simulink model "Schimmel_Evan_lab_4_model_single"  (R2020b)
settings: Solver=VariableStepAuto  StartTime=0.0  StopTime=tf  MaxStep=maxstep  RelTol=tol  AbsTol=tol
values from neighbouring files (symbols this model uses):
  C = mp*lpcg+mw*lwcg    (= 0.01745975)    [Schimmel_Evan_lab_4_script_double.m]    (also in Schimmel_Evan_lab_4_script_single.m)
  J = ((mp*lp^2)/12)+mp*(lpcg^2)+(1/2)*mw*((dw/2)^2)+mw*(lwcg^2)    (= 0.004070351125)    [Schimmel_Evan_lab_4_script_double.m]    (also in Schimmel_Evan_lab_4_script_single.m)
  k = g*(mp*lpcg+mw*lwcg)    (= 0.1712801475)    [Schimmel_Evan_lab_4_script_double.m]    (also in Schimmel_Evan_lab_4_script_single.m)
  omega0 = 0    [Schimmel_Evan_lab_4_script_double.m]    (also in Schimmel_Evan_lab_4_script_single.m)
  theta0 = 0    [Schimmel_Evan_lab_4_script_double.m]    (also in Schimmel_Evan_lab_4_script_single.m)
settings Model: Creator=schimmer  LastModifiedBy=schimmer
settings DataIOCC: SaveOutput=off  SignalLogging=off  DSMLogging=off  SaveTime=off  ReturnWorkspaceOutputs=off

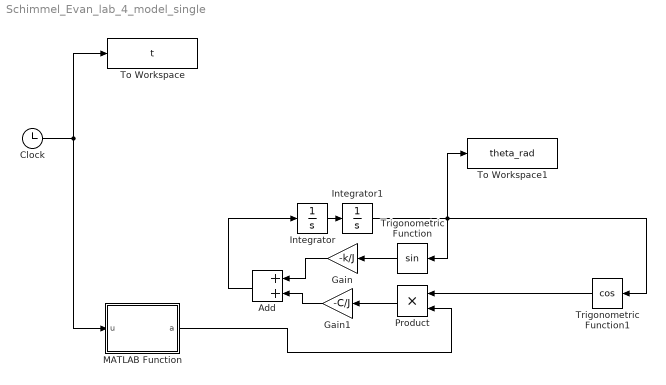
== system Schimmel_Evan_lab_4_model_single ==
  Add : Sum
  Clock : Clock
  Gain : Gain  Gain=-k/J
  Gain1 : Gain  Gain=-C/J
  Integrator : Integrator  InitialCondition=omega0
  Integrator1 : Integrator  InitialCondition=theta0
  MATLAB Function : MATLAB Function  TreatAsAtomicUnit=on
  Product : Product
  To Workspace : ToWorkspace  VariableName=t  SampleTime=-1
  To Workspace1 : ToWorkspace  VariableName=theta_rad  SampleTime=-1
  Trigonometric Function : Trigonometry
  Trigonometric Function1 : Trigonometry  Operator=cos
  wires:
  Integrator/1 -> Integrator1/1
  Clock/1 -> To Workspace/1, MATLAB Function/1(u)
  Trigonometric Function1/1 -> Product/1
  MATLAB Function/1(a) -> Product/2
  Integrator1/1 -> Trigonometric Function/1, To Workspace1/1, Trigonometric Function1/1
  Add/1 -> Integrator/1
  Trigonometric Function/1 -> Gain/1
  Product/1 -> Gain1/1
  Gain1/1 -> Add/2
  Gain/1 -> Add/1

== matlab function Schimmel_Evan_lab_4_model_single/MATLAB Function ==
  data: u input; a output
function a = fcn(u)
accel=(7194*exp(-43.5668*u+9.38)*(exp(-43.5668*u+9.38)-1))/((1+exp(-43.5668*u+9.38))^3);
a=accel/100;
